simulink model "SIMULACAO_PROJETO"  (R2022a)
settings: Solver=VariableStepAuto  StartTime=0.0  StopTime=20000  RelTol=1e-3
libraries: cstblocks x5
settings Model: Creator=allti  LastModifiedBy=allti

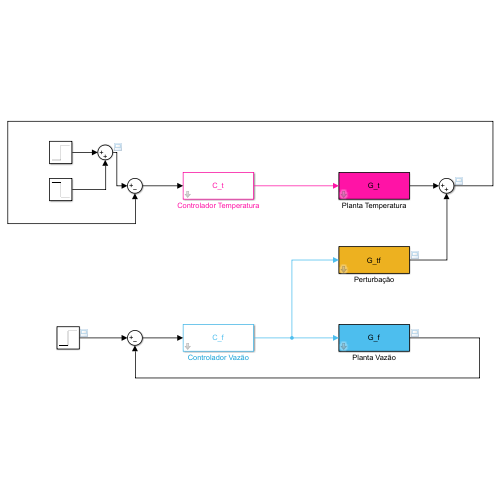
[thumbnail: Simulink's stored preview of the top-level diagram]
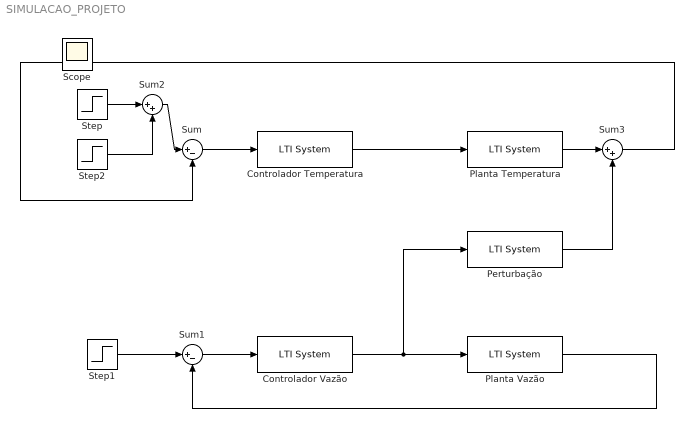
== system SIMULACAO_PROJETO ==
  Controlador Temperatura : cstblocks/LTI System  sys=C_t  IC=[]
  Controlador Vazão : cstblocks/LTI System  sys=C_f  IC=[]
  Perturbação : cstblocks/LTI System  sys=G_tf  IC=[]
  Planta Temperatura : cstblocks/LTI System  sys=G_t  IC=[]
  Planta Vazão : cstblocks/LTI System  sys=G_f  IC=[]
  Step : Step  After=20  SampleTime=0
  Step1 : Step  Time=6000  After=12  SampleTime=0
  Step2 : Step  Time=10000  After=-15  SampleTime=0
  Sum : Sum  Inputs=|+-
  Sum1 : Sum  Inputs=|+-
  Sum2 : Sum  Inputs=|++
  Sum3 : Sum  Inputs=|++
  Scope : Scope
  wires:
  Controlador Temperatura/1 -> Planta Temperatura/1
  Sum/1 -> Controlador Temperatura/1
  Controlador Vazão/1 -> Perturbação/1, Planta Vazão/1
  Step1/1 -> Sum1/1
  Sum1/1 -> Controlador Vazão/1
  Planta Vazão/1 -> Sum1/2
  Step/1 -> Sum2/1
  Step2/1 -> Sum2/2
  Sum2/1 -> Sum/1
  Planta Temperatura/1 -> Sum3/1
  Perturbação/1 -> Sum3/2
  Sum3/1 -> Sum/2
